simulink model "doublMassControl"  (R2016b)
settings: Solver=VariableStepAuto  StartTime=0.0  StopTime=0.3  FixedStep=2e-4  RelTol=1e-3
values from neighbouring files (symbols this model uses):
  denGc = denGc{1}    [doubleMassInit.m]
  denGp = [m1*m2 0 (m1+m2)*k 0 0]    [doubleMassInit.m]
  fs = 5000    [doubleMassInit.m]
  numGc = numGc{1}    [doubleMassInit.m]
  numGp = k    (= 355305758.439)    [doubleMassInit.m]
  Ts = 1/fs    (= 0.0002)    [doubleMassInit.m]
libraries: simulink x6, model_controller x2
settings Model: Creator=Dai Luyao  LastModifiedBy=Dai Luyao

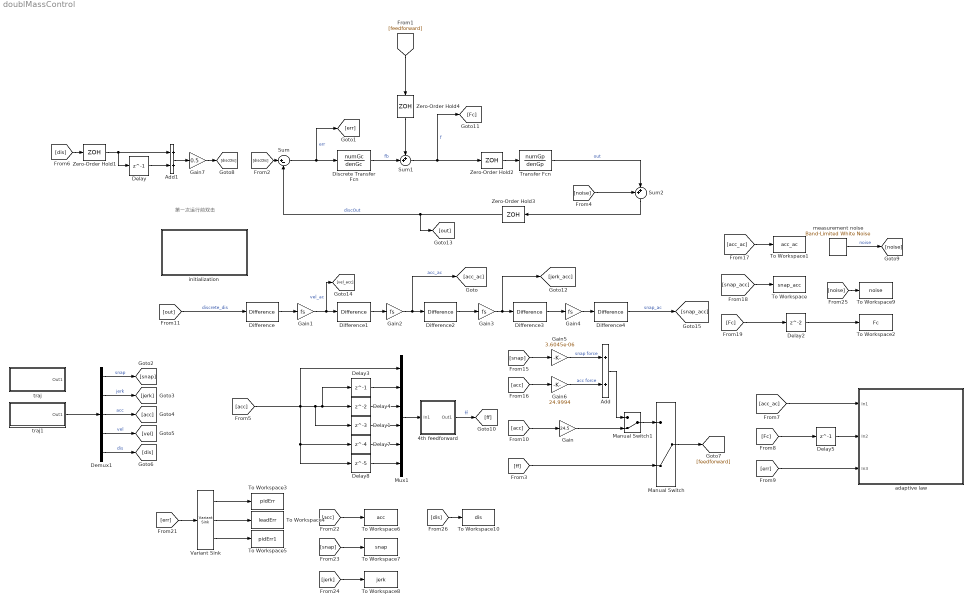
== system doublMassControl ==
  note: 第一次运行前双击
  4th feedforward : Subsystem
  Add : Sum
  Add1 : Sum
  Delay : Delay  DelayLength=1
  Delay1 : Delay  DelayLength=3
  Delay2 : Delay
  Delay3 : Delay  DelayLength=1
  Delay4 : Delay
  Delay5 : Delay  DelayLength=1
  Delay7 : Delay  DelayLength=4
  Delay8 : Delay  DelayLength=5
  Demux1 : Demux  Outputs=5
  Difference{,1..4} (5 alike) : simulink/Discrete/Difference  ICPrevInput=0.0  OutMin=[]  OutMax=[]  OutDataType=fixdt(1, 16)  OutScaling=2^-10  DoSatur=off
  Discrete Transfer Fcn : DiscreteTransferFcn  Numerator=numGc  Denominator=denGc  SampleTime=Ts
  Gain : Gain  Gain=24.5
  Gain{1..4} (4 alike) : Gain  Gain=fs
  Gain5 : Gain  Gain=3.6045e-06
  Gain6 : Gain  Gain=24.9994
  Gain7 : Gain  Gain=0.5
  Manual Switch : ManualSwitch  CurrentSetting=0
  Manual Switch1 : ManualSwitch  CurrentSetting=0
  Mux1 : Mux  Inputs=6
  Sum : Sum  Inputs=|+-
  Sum1 : Sum  Inputs=++|
  Sum2 : Sum  Inputs=++|
  To Workspace : ToWorkspace  VariableName=snap_acc  SampleTime=-1
  To Workspace1 : ToWorkspace  VariableName=acc_ac  SampleTime=-1
  To Workspace10 : ToWorkspace  VariableName=dis  SaveFormat=Structure With Time  SampleTime=-1
  To Workspace2 : ToWorkspace  VariableName=Fc  SampleTime=-1
  To Workspace3 : ToWorkspace  VariableName=pidErr  SaveFormat=Structure With Time  SampleTime=-1
  To Workspace4 : ToWorkspace  VariableName=leadErr  SaveFormat=Structure With Time  SampleTime=-1
  To Workspace5 : ToWorkspace  VariableName=pidErr1  SaveFormat=Structure With Time  SampleTime=-1
  To Workspace6 : ToWorkspace  VariableName=acc  SaveFormat=Structure With Time  SampleTime=-1
  To Workspace7 : ToWorkspace  VariableName=snap  SaveFormat=Structure With Time  SampleTime=-1
  To Workspace8 : ToWorkspace  VariableName=jerk  SaveFormat=Structure With Time  SampleTime=-1
  To Workspace9 : ToWorkspace  VariableName=noise  SaveFormat=Structure With Time  SampleTime=-1
  Transfer Fcn : TransferFcn  Numerator=numGp  Denominator=denGp
  Variant Sink : VariantSink
  Zero-Order Hold{1..4} (4 alike) : ZeroOrderHold  SampleTime=Ts
  "adaptive law " : Subsystem
  initialization : Subsystem
      settings: OpenFcn=doubleMassInit;  MoveFcn=edit doubleMassInit;
  measurement noise : simulink/Sources/Band-Limited White Noise  Cov=noisePower  Ts=Ts  seed=[23341]
  traj : Subsystem  BlockChoice=4th order traj
      link override 4th order traj: v=0.5  x=0.1  j=500
      settings: AttributesFormatString=%<BlockChoice>  TemplateBlock=model_controller/Profile Generators/traj  MemberBlocks=2th order traj,3rd order traj,4th order traj,step
  traj1 : Subsystem  BlockChoice=4th order traj
      link override 4th order traj: v=0.25
      settings: AttributesFormatString=%<BlockChoice>  TemplateBlock=model_controller/Profile Generators/traj  MemberBlocks=2th order traj,3rd order traj,4th order traj,step
  wires:
  Sum/1 -> Discrete Transfer Fcn/1, [err]  "err"
  Discrete Transfer Fcn/1 -> Sum1/2  "fb"
  Sum1/1 -> Zero-Order Hold2/1, [Fc]  "f"
  Difference1/1 -> Gain2/1
  Difference/1 -> Gain1/1
  Gain1/1 -> [vel_acc], Difference1/1  "vel_ac"
  [out] -> Difference/1  "discrete_dis"
  Mux1/1 -> 4th feedforward/1(In1)
  measurement noise/1 -> [noise]  "noise"
  Transfer Fcn/1 -> Sum2/2  "out"
  Demux1/1 -> [snap]  "snap"
  Demux1/2 -> [jerk]  "jerk"
  Demux1/3 -> [acc]  "acc"
  Demux1/4 -> [vel]  "vel"
  Demux1/5 -> [dis]  "dis"
  4th feedforward/1(Out1) -> [ff]  "ff"
  Difference2/1 -> Gain3/1
  Gain2/1 -> [acc_ac], Difference2/1  "acc_ac"
  Gain3/1 -> [jerk_acc], Difference3/1
  Gain4/1 -> Difference4/1
  Difference3/1 -> Gain4/1
  Difference4/1 -> [snap_acc]  "snap_ac"
  [acc] -> Gain/1
  [snap] -> Gain5/1
  [acc] -> Gain6/1
  Gain5/1 -> Add/1  "snap force"
  Gain6/1 -> Add/2  "acc force"
  Add/1 -> Manual Switch1/1
  Gain/1 -> Manual Switch1/2
  Manual Switch1/1 -> Manual Switch/1
  [ff] -> Manual Switch/2
  [acc_ac] -> To Workspace1/1
  [snap_acc] -> To Workspace/1
  [Fc] -> Delay2/1
  Delay2/1 -> To Workspace2/1
  Manual Switch/1 -> [feedforward]
  [err] -> Variant Sink/1
  Variant Sink/1 -> To Workspace3/1
  Variant Sink/2 -> To Workspace4/1
  Variant Sink/3 -> To Workspace5/1
  [acc] -> To Workspace6/1
  [snap] -> To Workspace7/1
  [jerk] -> To Workspace8/1
  [noise] -> To Workspace9/1
  [dis] -> To Workspace10/1
  Delay4/1 -> Mux1/3
  Delay3/1 -> Mux1/2
  Delay1/1 -> Mux1/4
  Delay8/1 -> Mux1/6
  Delay7/1 -> Mux1/5
  [acc] -> Delay8/1, Delay7/1, Mux1/1, Delay1/1, Delay3/1, Delay4/1
  [dis] -> Zero-Order Hold1/1
  Delay/1 -> Add1/2
  Zero-Order Hold1/1 -> Delay/1, Add1/1
  Add1/1 -> Gain7/1
  Zero-Order Hold2/1 -> Transfer Fcn/1
  Sum2/1 -> Zero-Order Hold3/1
  Zero-Order Hold3/1 -> [out], Sum/2  "discOut"
  Zero-Order Hold4/1 -> Sum1/1
  [err] -> "adaptive law "/3(In3)
  traj1/1(Out1) -> Demux1/1
  [acc_ac] -> "adaptive law "/1(In1)
  [feedforward] -> Zero-Order Hold4/1
  [noise] -> Sum2/1
  Gain7/1 -> [discDis]
  [discDis] -> Sum/1
  [Fc] -> Delay5/1
  Delay5/1 -> "adaptive law "/2(In2)

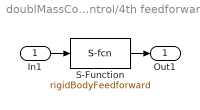
== system doublMassControl/4th feedforward ==
  In1 : Inport
  S-Function : S-Function  FunctionName=rigidBodyFeedforward  SFunctionDeploymentMode=off  EnableBusSupport=off
  Out1 : Outport
  wires:
  In1/1 -> S-Function/1
  S-Function/1 -> Out1/1

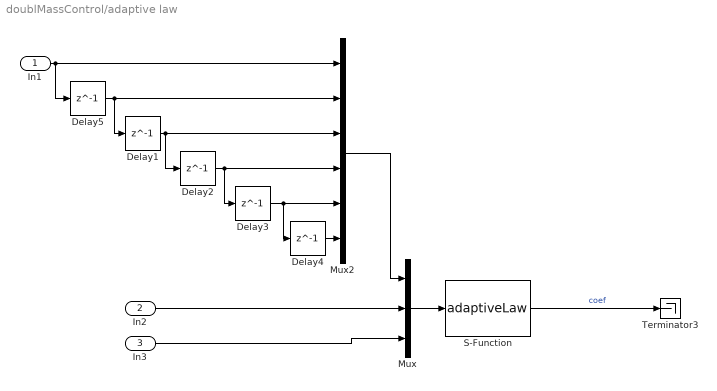
== system doublMassControl/adaptive law  ==
  In1 : Inport
  In2 : Inport  Port=2
  In3 : Inport  Port=3
  Delay{1..5} (5 alike) : Delay  DelayLength=1
  Mux : Mux  Inputs=3
  Mux2 : Mux  Inputs=6
  S-Function : S-Function  FunctionName=adaptiveLaw  Parameters=1  SFunctionDeploymentMode=off  EnableBusSupport=off
  Terminator3 : Terminator
  wires:
  Delay5/1 -> Delay1/1, Mux2/2
  Mux/1 -> S-Function/1
  In2/1 -> Mux/2
  In3/1 -> Mux/3
  S-Function/1 -> Terminator3/1  "coef"
  Mux2/1 -> Mux/1
  In1/1 -> Delay5/1, Mux2/1
  Delay1/1 -> Delay2/1, Mux2/3
  Delay2/1 -> Delay3/1, Mux2/4
  Delay3/1 -> Delay4/1, Mux2/5
  Delay4/1 -> Mux2/6

== system doublMassControl/initialization ==

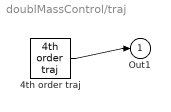
== system doublMassControl/traj ==
  4th order traj : model_controller/Profile Generators/4th order traj  t0=0  x=0.1  v=0.5  a=10  j=500  d=64000  Ts=0
  Out1 : Outport
  wires:
  4th order traj/1 -> Out1/1

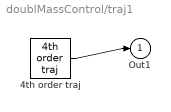
== system doublMassControl/traj1 ==
  4th order traj : model_controller/Profile Generators/4th order traj  t0=0  x=0.06  v=0.25  a=10  j=800  d=64000  Ts=0
  Out1 : Outport
  wires:
  4th order traj/1 -> Out1/1
